simulink model "aerosonde_uncontrolled"  (Simulink 7.7)
settings: Solver=ode3  StartTime=0.0  StopTime=5  FixedStep=20e-3  RelTol=1e-6
values from neighbouring files (symbols this model uses):
  aerosonde = aerosonde_data    [aerosonde_initialize.m]    (also in aerosonde_trimlin.m)
  control_0 = [flap ... (first row only)    [aerosonde_initialize.m]    (also in aerosonde_trimlin.m = [0;utrim;13;1])
  euler_0 = [theta_trim; 0; 0]    [aerosonde_initialize.m]    (also in aerosonde_trimlin.m = xtrim(11:13))
  fuel_0 = 2    [aerosonde_initialize.m]    (also in aerosonde_trimlin.m = xtrim(10))
  Omega_0 = 5000*pi/30    (= 523.598775598)    [aerosonde_initialize.m]    (also in aerosonde_trimlin.m = xtrim(14))
  position_0 = [0; 0; -h_trim]    [aerosonde_initialize.m]
  rates_0 = [0; q_trim ; 0]    [aerosonde_initialize.m]    (also in aerosonde_trimlin.m = xtrim(7:9))
  velocity_0 = [23; 0; 0]    [aerosonde_initialize.m]    (also in aerosonde_trimlin.m = xtrim(1:3))
undefined symbols (not defined in the file or in its folder): F, Light, MIL
libraries: aerolibasang x3, aerolibbdyn x3, simulink_extras x3, aerolibwind2 x3, aerolibfltsims x2, aerolibadyn x1, aerolibtransform2 x1, aerolib6dof2 x1, aerolibutil x1, aerolibatmos2 x1
(part 2 of 2)

== system aerosonde_uncontrolled/Aerosonde UAV Dynamics/Propulsion System/Piston Engine/Altitude correction  for  Power ==
  note: Altitude correction for Power
  T : Inport
  Math Function : Math  Operator=sqrt  SaturateOnIntegerOverflow=on
  Product of Elements : Product  Inputs=/
  "Sea-level temperature " : Gain  Gain=TSL  SaturateOnIntegerOverflow=on  OutDataTypeStr=Inherit: Same as input  ParamDataTypeStr=Inherit: Same as input
  Power correction : Outport
  wires:
  T/1 -> Product of Elements/1
  Math Function/1 -> Power correction/1
  "Sea-level temperature "/1 -> Math Function/1
  Product of Elements/1 -> "Sea-level temperature "/1

== system aerosonde_uncontrolled/Aerosonde UAV Dynamics/Propulsion System/Piston Engine/Intake ==
  Thr : Inport  OutDataTypeStr=double  PortDimensions=1
  P_atm : Inport  Port=2  OutDataTypeStr=double  PortDimensions=1
  Get MAP : Product  SaturateOnIntegerOverflow=on  InputSameDT=on  OutDataTypeStr=Inherit: Same as first input
  MAP min : Constant  Value=as.MAPmin
  Saturation : Saturate  UpperLimit=inf  LowerLimit=as.MAPmin
  Sum : Sum  Inputs=|+-  SaturateOnIntegerOverflow=on  InputSameDT=on  OutDataTypeStr=Inherit: Same as first input
  Sum1 : Sum  Inputs=|++  SaturateOnIntegerOverflow=on  InputSameDT=on  OutDataTypeStr=Inherit: Same as first input
  kPa : Gain  Gain=1/1000  SaturateOnIntegerOverflow=on  OutDataTypeStr=Inherit: Same as input  ParamDataTypeStr=Inherit: Same as input
  MAP : Outport
  wires:
  Saturation/1 -> MAP/1
  P_atm/1 -> kPa/1
  Thr/1 -> Get MAP/1
  MAP min/1 -> Sum/2, Sum1/2
  kPa/1 -> Sum/1
  Sum/1 -> Get MAP/2
  Get MAP/1 -> Sum1/1
  Sum1/1 -> Saturation/1
